simulink library "UXFD_Lib"  (R2016b)
settings: Solver=ode45  StartTime=0.0  StopTime=10.0  RelTol=1e-3  EnableMultiTasking=on
undefined symbols (not defined in the file): BreakpointData, BreakpointData1, BreakpointData2, BreakpointData_One_A, BreakpointData_Two_A, E2E_P01DataIDMode, E2E_P01ReceiverStatusType, EnumClass, iBit, initalValue, No_Runnable_Period, ObB_EidBsgStDerat_C, p_OVERRIDE_MASTER_SWITCH, SlDemoSign, SwitchOff_P, SwitchOn_P, Table, TableData_M, VCCTi33, VSysD_FidVehDerat1_C
libraries: simulink x28, CCMLib x11, UXFD_Lib x8, canmsglib x2, PTCC_Lib x1, hdlsllib x1
(part 7 of 7)

== system UXFD_Lib/Custom/CAN/CanHex2Signed/signal_conditioning ==
  note: 判断输入的BitLength是否（0<u1<=32bit）;
      | 并向下取整。
  In1 : Inport
  Constant1 : Constant  Value=0  OutDataTypeStr=single
      settings: CopyFcn=set_param(gcbh,'ShowName','off');
  Constant2 : Constant  Value=32  OutDataTypeStr=single
      settings: CopyFcn=set_param(gcbh,'ShowName','off');
  Constant4 : Constant  Value=32  OutDataTypeStr=single
      settings: CopyFcn=set_param(gcbh,'ShowName','off');
  Constant7 : Constant  Value=0  OutDataTypeStr=single
      settings: CopyFcn=set_param(gcbh,'ShowName','off');
  Floor : Subsystem  mask(GL_Floor){}
      mask help: Floor block rounds the input variable to the nearest integer towards minus infinity.
      mask init:
      | set_param(gcb,'LinkStatus','none');
      settings: CopyFcn=set_param(gcbh,'ShowName','off');
      mask Display: text(0.1,0.5, 'Floor')
  Relational Operator1 : RelationalOperator  Operator=<  OutDataTypeStr=boolean  RndMeth=Nearest
  Relational Operator2 : RelationalOperator  Operator=>  OutDataTypeStr=boolean  RndMeth=Nearest
  Switch : Switch  Criteria=u2 > Threshold
  Switch1 : Switch  Criteria=u2 > Threshold
  BitLength_BeUsed : Outport
  wires:
  Floor/1(Out1) -> Switch1/1
  Relational Operator2/1 -> Switch/2
  Constant1/1 -> Relational Operator2/2
  Relational Operator1/1 -> Switch1/2
  Switch/1 -> Floor/1(In1), Relational Operator1/1
  Constant4/1 -> Relational Operator1/2
  Constant2/1 -> Switch1/3
  Switch1/1 -> BitLength_BeUsed/1
  Constant7/1 -> Switch/3
  In1/1 -> Relational Operator2/1, Switch/1

== system UXFD_Lib/Custom/CAN/CanHex2Signed/value<0 ==
  hex : Inport
  2^n : Inport  Port=2  OutDataTypeStr=single
  Action Port : ActionPort
  Add : Sum  Inputs=+-
      settings: CopyFcn=set_param(gcbh,'ShowName','off');
  Gain1 : Gain  OutDataTypeStr=single
      settings: CopyFcn=set_param(gcbh,'ShowName','off');
  Gain8 : Gain  OutDataTypeStr=single
      settings: CopyFcn=set_param(gcbh,'ShowName','off');
  Out1 : Outport
  wires:
  Gain1/1 -> Add/2
  2^n/1 -> Gain1/1
  Gain8/1 -> Out1/1
  Add/1 -> Gain8/1
  hex/1 -> Add/1

== system UXFD_Lib/Custom/CAN/CanHex2Signed/value>0 ==
  hex : Inport
  Action Port : ActionPort
  Gain9 : Gain  OutDataTypeStr=single
      settings: CopyFcn=set_param(gcbh,'ShowName','off');
  Out1 : Outport
  wires:
  Gain9/1 -> Out1/1
  hex/1 -> Gain9/1

== system UXFD_Lib/Custom/Diagnose/Dem_SetEventStatus/Dem_SetEventStatus_Enable ==
  EventID : Inport
  EveSt : Inport  Port=2
  Enable : EnablePort
  Dem_SetEventStatus_Asw : S-Function  FunctionName=Dem_SetEventStatus_Asw_SF  SFunctionDeploymentMode=off  EnableBusSupport=off  mask(Legacy Function){SFunctionSpec=void Dem_SetEventStatus_Asw(uint16 u1, uint8 u2), ShowSpec=on}
      mask prompts: ShowSpec "Display function specification"
      mask help:
      | This block allows you to call the legacy functions specified by the following Legacy Code Tool definition:
      | def.SFunctionName = 'Dem_SetEventStatus_Asw_SF';
      | def.OutputFcnSpec = 'void Dem_SetEventStatus_Asw(uint16 u1, uint8 u2)';
      | def.HeaderFiles = {'Dem.h'};
      | def.SourceFiles = {'Dem.c'};
      mask Help: <p>This block was generated automatically by the Legacy Code Tool. For detailed help on this tool, call<a href="matlab:legacy_code('help')"> legacy_code('help')</a>.</p>
      mask Callback ShowSpec:
      | if strcmp(get_param(gcbh, 'ShowSpec'), 'on')
      |   set_param(gcbh, 'MaskDisplay', sprintf('fprintf(''%s'');', get_param(gcbh, 'SFunctionSpec')));
      | else
      |   set_param(gcbh, 'MaskDisplay', sprintf('fprintf(''%s'');', get_param(gcbh, 'FunctionName')));
      | end
      mask Display: fprintf('void Dem_SetEventStatus_Asw(uint16 u1, uint8 u2)');
  wires:
  EveSt/1 -> Dem_SetEventStatus_Asw/2
  EventID/1 -> Dem_SetEventStatus_Asw/1

== system UXFD_Lib/Standard/Discrete dynamics/BumplessRateTransfer/LogicalSwitch1 ==
  In1 : Inport
  In2 : Inport  Port=2
  In3 : Inport  Port=3
  Switch : Switch  Criteria=u2 > Threshold  Threshold=0.5
  Out1 : Outport
  wires:
  In1/1 -> Switch/1
  In3/1 -> Switch/2
  In2/1 -> Switch/3
  Switch/1 -> Out1/1

== system UXFD_Lib/Standard/Discrete dynamics/BumplessRateTransfer/RateLimit ==
  In1 : Inport
  dr : Inport  Port=2
  df : Inport  Port=3
  Abs : Abs
  Add : Sum  Inputs=+-
  Add1 : Sum
  MinMax : MinMax  Function=max  Inputs=2
  MinMax1 : MinMax  Inputs=2
  Product : Product
  Product1 : Product
  Subsystem1 : Subsystem
      mask help:
      | this block use for the situation when the first run use the Initail Value , after the first run , use the CalValue.
      | output is the Initial Value when first run ; otherwise is the calValue.
      mask Display: dpoly([0 0 1], [0 1 0], 'z')
  ts : DataStoreRead  DataStoreName=ts
  y : Outport
  wires:
  In1/1 -> Subsystem1/1(InitialValue), MinMax/1
  Add1/1 -> MinMax1/2
  dr/1 -> Product1/2
  MinMax1/1 -> Subsystem1/2(CalValue), y/1
  Product1/1 -> Add1/2
  MinMax/1 -> MinMax1/1
  Add/1 -> MinMax/2
  Product/1 -> Abs/1
  df/1 -> Product/2
  ts/1 -> Product1/1, Product/1
  Abs/1 -> Add/2
  Subsystem1/1(Output) -> Add1/1, Add/1

== system UXFD_Lib/Standard/Discrete dynamics/BumplessTransfer/LPF1_pole1 ==
  u : Inport
  tc : Inport  Port=2
  Add : Sum  Inputs=-+
  Add1 : Sum
  Constant : Constant  Value=1e-6  OutDataTypeStr=single
  Divide : Product  Inputs=*/
  MinMax : MinMax  Function=max  Inputs=3
  Product : Product
  Subsystem1 : Subsystem
      mask help:
      | this block use for the situation when the first run use the Initail Value , after the first run , use the CalValue.
      | output is the Initial Value when first run ; otherwise is the calValue.
      mask Display: dpoly([0 0 1], [0 1 0], 'z')
  ts : DataStoreRead  DataStoreName=ts
  y : Outport
  wires:
  Add1/1 -> Subsystem1/2(CalValue), y/1
  u/1 -> Subsystem1/1(InitialValue), Add/2
  Add/1 -> Product/1
  MinMax/1 -> Divide/2
  tc/1 -> MinMax/2
  ts/1 -> Divide/1, MinMax/1
  Divide/1 -> Product/2
  Subsystem1/1(Output) -> Add/1, Add1/1
  Product/1 -> Add1/2
  Constant/1 -> MinMax/3

== system UXFD_Lib/Standard/Discrete dynamics/BumplessTransfer/LogicalSwitch1 ==
  In1 : Inport
  In2 : Inport  Port=2
  In3 : Inport  Port=3
  Switch : Switch  Criteria=u2 > Threshold  Threshold=0.5
  Out1 : Outport
  wires:
  In1/1 -> Switch/1
  In3/1 -> Switch/2
  In2/1 -> Switch/3
  Switch/1 -> Out1/1

== system UXFD_Lib/Standard/Discrete dynamics/DLPF1_pole_v2/LogicalSwitch1 ==
  In1 : Inport
  In2 : Inport  Port=2
  In3 : Inport  Port=3
  Switch : Switch  Criteria=u2 > Threshold  Threshold=0.5
  Out1 : Outport
  wires:
  In1/1 -> Switch/1
  In3/1 -> Switch/2
  In2/1 -> Switch/3
  Switch/1 -> Out1/1

== system UXFD_Lib/Standard/Discrete dynamics/HysteresisFilter/Saturation1 ==
  u : Inport
  U : Inport  Port=2
  L : Inport  Port=3
  MinMax : MinMax  Inputs=2
  MinMax1 : MinMax  Function=max  Inputs=2
  y : Outport
  wires:
  L/1 -> MinMax1/2
  MinMax1/1 -> y/1
  u/1 -> MinMax/2
  U/1 -> MinMax/1
  MinMax/1 -> MinMax1/1

== system UXFD_Lib/Standard/Discrete dynamics/LPF1_discreteReset/LogicalSwitch1 ==
  In1 : Inport
  In3 : Inport  Port=2
  In2 : Inport  Port=3
  Switch : Switch  Criteria=u2 ~= 0  Threshold=0.5  SaturateOnIntegerOverflow=on  InputSameDT=on  mask(TL_Switch){data={'logdata',{'maxnumvals',4096,'plotchannels',[]},'output',{'type','Float32'},'date',735300.29228125}}
      settings: CopyFcn=if exist('tl_reset_reviewflag','file')==2,tl_reset_reviewflag(gcbh);end  DeleteFcn=if exist('delete_tlblock','file')==2,delete_tlblock(gcbh);end  NameChangeFcn=if exist('rename_tlblock','file')==2,rename_tlblock(gcbh);end  OpenFcn=if exist('tl_open_blockdlg','file')==2,tl_open_blockdlg(gcbh);else,open_system(gcbh,'parameter');end
      mask Help: eval(['if exist(''tl_online_help'',''file'') == 2, tl_online_help(''Topic'',''TL_Switch''),else, web([''jar:file:///'',matlabroot,''/help/toolbox/simulink/help.jar!/slref/' lower(get_param(gcbh,'Blocktype')) '.html''], ''-helpbrowser''),end'])
      mask Display: plot([-0.05, 1.05, NaN, -0.05, 1.05],[.01, .01, NaN, .99, .99])
  Out1 : Outport
  wires:
  In1/1 -> Switch/1
  In2/1 -> Switch/2
  In3/1 -> Switch/3
  Switch/1 -> Out1/1

== system UXFD_Lib/Standard/Math/Floor/mod1 ==
  In1 : Inport
  In2 : Inport  Port=2
  Mod : Math  Operator=mod  SaturateOnIntegerOverflow=on
  Out1 : Outport
  wires:
  In1/1 -> Mod/1
  Mod/1 -> Out1/1
  In2/1 -> Mod/2

== system UXFD_Lib/Standard/Math/Interpolation/Safe_Divide ==
  In3 : Inport
  In2 : Inport  Port=2
  In1 : Inport  Port=3
  Constant : Constant  Value=0  OutDataTypeStr=Inherit: Inherit via back propagation
  Gain : Gain  Gain=-1
  LogicalSwitch : Subsystem  mask(PAG_Switch_LV1.6_BV2){}
      mask help:
      | Pass through input 1 when input 3 is true;
      | otherwise, pass through input 2
      mask Display:
      | plot([-0.1 0.2 0.2], [0.85 0.85 0.75])
      | plot([-0.1 0.2 0.2], [0.5 0.5 0.6])
      | plot([0.8 1.1], [0.5 0.5])
      | plot([0.15 0.8], [0.6 0.5])
      | plot([-0.1 0.5 0.5], [0.15 0.15 0.6])
  Max : MinMax  Function=max  Inputs=2
  MinMax : MinMax  Inputs=2
  Product1 : Product  Inputs=*/
  Relational Operator : RelationalOperator  Operator=<  OutDataTypeStr=boolean  RndMeth=Nearest
  Out1 : Outport
  wires:
  Constant/1 -> Relational Operator/2
  Relational Operator/1 -> LogicalSwitch/3(In3)
  MinMax/1 -> LogicalSwitch/1(In1)
  In1/1 -> Gain/1, Max/1
  In2/1 -> Relational Operator/1, Max/2, MinMax/1
  Max/1 -> LogicalSwitch/2(In2)
  In3/1 -> Product1/1
  Product1/1 -> Out1/1
  Gain/1 -> MinMax/2
  LogicalSwitch/1(Out1) -> Product1/2

== system UXFD_Lib/Standard/Math/LimitInterpolation/Safe_Divide ==
  In3 : Inport
  In2 : Inport  Port=2
  In1 : Inport  Port=3
  Constant : Constant  Value=0  OutDataTypeStr=Inherit: Inherit via back propagation
  Gain : Gain  Gain=-1
  LogicalSwitch : Subsystem  mask(PAG_Switch_LV1.6_BV2){}
      mask help:
      | Pass through input 1 when input 3 is true;
      | otherwise, pass through input 2
      mask Display:
      | plot([-0.1 0.2 0.2], [0.85 0.85 0.75])
      | plot([-0.1 0.2 0.2], [0.5 0.5 0.6])
      | plot([0.8 1.1], [0.5 0.5])
      | plot([0.15 0.8], [0.6 0.5])
      | plot([-0.1 0.5 0.5], [0.15 0.15 0.6])
  Max : MinMax  Function=max  Inputs=2
  MinMax : MinMax  Inputs=2
  Product1 : Product  Inputs=*/
  Relational Operator : RelationalOperator  Operator=<  OutDataTypeStr=boolean  RndMeth=Nearest
  Out1 : Outport
  wires:
  Constant/1 -> Relational Operator/2
  Relational Operator/1 -> LogicalSwitch/3(In3)
  MinMax/1 -> LogicalSwitch/1(In1)
  In1/1 -> Gain/1, Max/1
  In2/1 -> Relational Operator/1, Max/2, MinMax/1
  Max/1 -> LogicalSwitch/2(In2)
  In3/1 -> Product1/1
  Product1/1 -> Out1/1
  Gain/1 -> MinMax/2
  LogicalSwitch/1(Out1) -> Product1/2

== system UXFD_Lib/Standard/Math/LimitInterpolation/Saturation ==
  u : Inport
  U : Inport  Port=2
  L : Inport  Port=3
  MinMax : MinMax  Inputs=2
  MinMax1 : MinMax  Function=max  Inputs=2
  y : Outport
  wires:
  MinMax/1 -> MinMax1/1
  U/1 -> MinMax/1
  u/1 -> MinMax/2
  MinMax1/1 -> y/1
  L/1 -> MinMax1/2

== system UXFD_Lib/Standard/Math/Round/mod ==
  In1 : Inport
  In2 : Inport  Port=2
  mod : Subsystem  mask(GL_Mod_1.0){}
      mask help: Signed remainder after division.
      mask Display: disp('mod')
  Out1 : Outport
  wires:
  In1/1 -> mod/1(In1)
  mod/1(Out1) -> Out1/1
  In2/1 -> mod/2(In2)

== system UXFD_Lib/Standard/Math/Safe_Divide/LogicalSwitch ==
  In1 : Inport
  In2 : Inport  Port=2
  In3 : Inport  Port=3
  Switch : Switch  Criteria=u2 ~= 0  Threshold=1  OutDataTypeStr=Inherit: Inherit via back propagation  RndMeth=Round  SaturateOnIntegerOverflow=on  InputSameDT=on
      settings: AttributesFormatString=%<Criteria>  CopyFcn=set_param(gcbh,'ShowName','off');
  Out1 : Outport
  wires:
  In1/1 -> Switch/1
  In3/1 -> Switch/2
  In2/1 -> Switch/3
  Switch/1 -> Out1/1

== system UXFD_Lib/Autosar/E2E_P01_Check/E2E_Check/E2E_Check/Data_ID_218 ==
  CheckSum : Inport
  RollingCounter : Inport  Port=2
  AccrPedlNotCmpl_Psd : Inport  Port=3
  AccrPedlNotCmpl_PsdSts : Inport  Port=4
  Data Type Conversion{1..2,4..5} (4 alike) : DataTypeConversion  OutDataTypeStr=uint8
  Data Type Conversion6 : DataTypeConversion
  Mux2 : Mux
  Data_pu8 : Outport
  wires:
  Data Type Conversion4/1 -> Mux2/3
  Data Type Conversion5/1 -> Mux2/4
  Mux2/1 -> Data Type Conversion6/1
  Data Type Conversion6/1 -> Data_pu8/1
  RollingCounter/1 -> Data Type Conversion1/1
  CheckSum/1 -> Data Type Conversion2/1
  AccrPedlNotCmpl_PsdSts/1 -> Data Type Conversion5/1
  AccrPedlNotCmpl_Psd/1 -> Data Type Conversion4/1
  Data Type Conversion1/1 -> Mux2/2
  Data Type Conversion2/1 -> Mux2/1

== system UXFD_Lib/Autosar/E2E_P01_Check/E2E_Check/E2E_Check/E2E_Config_ID_218 ==
  DataLength : Inport
  DataID : Inport  Port=2
  BusCreator2 : BusCreator  Inputs=6  OutDataTypeStr=Bus: E2E_P01ConfigType  NonVirtualBus=on
      settings: CopyFcn=set_param(gcbh,'ShowName','off');  InheritFromInputs=off
  CRCOffset : Constant  Value=0  OutDataTypeStr=uint16
  CounterOffset : Constant  Value=8  OutDataTypeStr=uint16
  DataIDMode : simulink/Sources/Enumerated Constant  OutDataTypeStr=Enum: E2E_P01DataIDMode  Value=E2E_P01DataIDMode.E2E_P01_DATAID_BOTH  SampleTime=inf
  MaxDeltaCounterInit : Constant  Value=14  OutDataTypeStr=uint8
  E2E_Config_ID_218 : Outport
  wires:
  CounterOffset/1 -> BusCreator2/6
  DataLength/1 -> BusCreator2/1
  MaxDeltaCounterInit/1 -> BusCreator2/4
  BusCreator2/1 -> E2E_Config_ID_218/1
  CRCOffset/1 -> BusCreator2/5
  DataID/1 -> BusCreator2/2
  DataIDMode/1 -> BusCreator2/3

== system UXFD_Lib/Autosar/E2E_P01_Check/E2E_Check/E2E_Check/E2E_P01Check_S ==
  ConfigType : Inport
  ReceiverStateType : Inport  Port=2
  Data_pu8 : Inport  Port=3
  S-Function : S-Function  FunctionName=E2E_P01Check_S  SFunctionDeploymentMode=off  EnableBusSupport=off
  Std_ReturnType : Outport
  wires:
  S-Function/1 -> Std_ReturnType/1
  Data_pu8/1 -> S-Function/3
  ConfigType/1 -> S-Function/1
  ReceiverStateType/1 -> S-Function/2

== system UXFD_Lib/Autosar/E2E_P01_Check/E2E_Check/E2E_Check/E2E_P01ReceiverID_218 ==
  AccrPedlNotCmpl_IsUpdated : Inport  OutDataTypeStr=boolean
  Status : Inport  Port=2
  BusCreator3 : BusCreator  Inputs=6  OutDataTypeStr=Bus: E2E_P01ReceiverStateType  NonVirtualBus=on
      settings: CopyFcn=set_param(gcbh,'ShowName','off');  InheritFromInputs=off
  LastValidCounter : Constant  Value=0  OutDataTypeStr=uint8
  LostData : Constant  Value=0  OutDataTypeStr=uint8
  MaxDeltaCounter : Constant  Value=0  OutDataTypeStr=uint8
  WaitForFirstData : Constant  OutDataTypeStr=boolean
  E2E_P01ReceiverState : Outport
  wires:
  LastValidCounter/1 -> BusCreator3/1
  WaitForFirstData/1 -> BusCreator3/3
  MaxDeltaCounter/1 -> BusCreator3/2
  LostData/1 -> BusCreator3/5
  BusCreator3/1 -> E2E_P01ReceiverState/1
  AccrPedlNotCmpl_IsUpdated/1 -> BusCreator3/4
  Status/1 -> BusCreator3/6

== system UXFD_Lib/Custom/CAN/CanHex2Signed/signal_conditioning/Floor ==
  In1 : Inport
  Add : Sum  Inputs=+-
  Constant : Constant  OutDataTypeStr=single
  mod1 : Subsystem  mask(GL_Mod_1.0){}
      mask help: Signed remainder after division.
      mask Display: disp('mod')
  Out1 : Outport
  wires:
  Constant/1 -> mod1/2(In2)
  Add/1 -> Out1/1
  In1/1 -> mod1/1(In1), Add/1
  mod1/1(Out1) -> Add/2

== system UXFD_Lib/Standard/Discrete dynamics/BumplessRateTransfer/RateLimit/Subsystem1 ==
  InitialValue : Inport
  CalValue : Inport  Port=2
  Constant12 : Constant  Value=0
      settings: CopyFcn=set_param(gcbh,'ShowName','off');
  ESubsystem : Subsystem  TreatAsAtomicUnit=on
      mask init:
      | set_param(gcb, 'LinkStatus', 'none');
      mask Display: disp(' ');
  Relational Operator10 : RelationalOperator  Operator===  OutDataTypeStr=boolean  RndMeth=Nearest
      settings: CopyFcn=set_param(gcbh,'ShowName','off');
  Switch1 : Switch  Criteria=u2 ~= 0  Threshold=1  OutDataTypeStr=Inherit: Inherit via back propagation  RndMeth=Round  SaturateOnIntegerOverflow=on  InputSameDT=on
      settings: AttributesFormatString=%<Criteria>  CopyFcn=set_param(gcbh,'ShowName','off');
  Unit Delay : UnitDelay  SampleTime=-1
      settings: CopyFcn=set_param(gcbh,'ShowName','off');
  Unit Delay1 : UnitDelay  SampleTime=-1
      settings: CopyFcn=set_param(gcbh,'ShowName','off');
  Output : Outport
  wires:
  Constant12/1 -> Relational Operator10/2
  ESubsystem/1(Out1) -> Unit Delay/1
  Unit Delay/1 -> Relational Operator10/1
  Relational Operator10/1 -> Switch1/2, ESubsystem/Enable
  InitialValue/1 -> Switch1/1
  CalValue/1 -> Unit Delay1/1
  Switch1/1 -> Output/1
  Unit Delay1/1 -> Switch1/3

== system UXFD_Lib/Standard/Discrete dynamics/BumplessTransfer/LPF1_pole1/Subsystem1 ==
  InitialValue : Inport
  CalValue : Inport  Port=2
  Constant12 : Constant  Value=0
      settings: CopyFcn=set_param(gcbh,'ShowName','off');
  ESubsystem : Subsystem  TreatAsAtomicUnit=on
      mask init:
      | set_param(gcb, 'LinkStatus', 'none');
      mask Display: disp(' ');
  Relational Operator10 : RelationalOperator  Operator===  OutDataTypeStr=boolean  RndMeth=Nearest
      settings: CopyFcn=set_param(gcbh,'ShowName','off');
  Switch1 : Switch  Criteria=u2 ~= 0  Threshold=1  OutDataTypeStr=Inherit: Inherit via back propagation  RndMeth=Round  SaturateOnIntegerOverflow=on  InputSameDT=on
      settings: AttributesFormatString=%<Criteria>  CopyFcn=set_param(gcbh,'ShowName','off');
  Unit Delay : UnitDelay  SampleTime=-1
      settings: CopyFcn=set_param(gcbh,'ShowName','off');
  Unit Delay1 : UnitDelay  SampleTime=-1
      settings: CopyFcn=set_param(gcbh,'ShowName','off');
  Output : Outport
  wires:
  Constant12/1 -> Relational Operator10/2
  ESubsystem/1(Out1) -> Unit Delay/1
  Unit Delay/1 -> Relational Operator10/1
  Relational Operator10/1 -> Switch1/2, ESubsystem/Enable
  InitialValue/1 -> Switch1/1
  CalValue/1 -> Unit Delay1/1
  Switch1/1 -> Output/1
  Unit Delay1/1 -> Switch1/3

== system UXFD_Lib/Standard/Math/Interpolation/Safe_Divide/LogicalSwitch ==
  In1 : Inport
  In2 : Inport  Port=2
  In3 : Inport  Port=3
  Switch : Switch  Threshold=0.5  SaturateOnIntegerOverflow=on  InputSameDT=on  mask(TL_Switch){data={'logdata',{'maxnumvals',4096,'plotchannels',[]},'output',{'type','Float32'},'date',735300.29223627318}}
      settings: CopyFcn=if exist('tl_reset_reviewflag','file')==2,tl_reset_reviewflag(gcbh);end  DeleteFcn=if exist('delete_tlblock','file')==2,delete_tlblock(gcbh);end  NameChangeFcn=if exist('rename_tlblock','file')==2,rename_tlblock(gcbh);end  OpenFcn=if exist('tl_open_blockdlg','file')==2,tl_open_blockdlg(gcbh);else,open_system(gcbh,'parameter');end
      mask Help: eval(['if exist(''tl_online_help'',''file'') == 2, tl_online_help(''Topic'',''TL_Switch''),else, web([''jar:file:///'',matlabroot,''/help/toolbox/simulink/help.jar!/slref/' lower(get_param(gcbh,'Blocktype')) '.html''], ''-helpbrowser''),end'])
      mask Display: plot([-0.05, 1.05, NaN, -0.05, 1.05],[.01, .01, NaN, .99, .99])
  Out1 : Outport
  wires:
  Switch/1 -> Out1/1
  In2/1 -> Switch/3
  In3/1 -> Switch/2
  In1/1 -> Switch/1

== system UXFD_Lib/Standard/Math/LimitInterpolation/Safe_Divide/LogicalSwitch ==
  In1 : Inport
  In2 : Inport  Port=2
  In3 : Inport  Port=3
  Switch : Switch  Threshold=0.5  SaturateOnIntegerOverflow=on  InputSameDT=on  mask(TL_Switch){data={'logdata',{'maxnumvals',4096,'plotchannels',[]},'output',{'type','Float32'},'date',735300.29223627318}}
      settings: CopyFcn=if exist('tl_reset_reviewflag','file')==2,tl_reset_reviewflag(gcbh);end  DeleteFcn=if exist('delete_tlblock','file')==2,delete_tlblock(gcbh);end  NameChangeFcn=if exist('rename_tlblock','file')==2,rename_tlblock(gcbh);end  OpenFcn=if exist('tl_open_blockdlg','file')==2,tl_open_blockdlg(gcbh);else,open_system(gcbh,'parameter');end
      mask Help: eval(['if exist(''tl_online_help'',''file'') == 2, tl_online_help(''Topic'',''TL_Switch''),else, web([''jar:file:///'',matlabroot,''/help/toolbox/simulink/help.jar!/slref/' lower(get_param(gcbh,'Blocktype')) '.html''], ''-helpbrowser''),end'])
      mask Display: plot([-0.05, 1.05, NaN, -0.05, 1.05],[.01, .01, NaN, .99, .99])
  Out1 : Outport
  wires:
  Switch/1 -> Out1/1
  In2/1 -> Switch/3
  In3/1 -> Switch/2
  In1/1 -> Switch/1

== system UXFD_Lib/Standard/Math/Round/mod/mod ==
  In1 : Inport
  In2 : Inport  Port=2
  Mod : Math  Operator=mod  SaturateOnIntegerOverflow=on
  Out1 : Outport
  wires:
  In1/1 -> Mod/1
  Mod/1 -> Out1/1
  In2/1 -> Mod/2

== system UXFD_Lib/Custom/CAN/CanHex2Signed/signal_conditioning/Floor/mod1 ==
  In1 : Inport
  In2 : Inport  Port=2
  Mod : Math  Operator=mod  SaturateOnIntegerOverflow=on
  Out1 : Outport
  wires:
  In1/1 -> Mod/1
  Mod/1 -> Out1/1
  In2/1 -> Mod/2

== system UXFD_Lib/Standard/Discrete dynamics/BumplessRateTransfer/RateLimit/Subsystem1/ESubsystem ==
  Enable_Name : EnablePort
  Constant10 : Constant
      settings: CopyFcn=set_param(gcbh,'ShowName','off');
  Out1 : Outport
  wires:
  Constant10/1 -> Out1/1

== system UXFD_Lib/Standard/Discrete dynamics/BumplessTransfer/LPF1_pole1/Subsystem1/ESubsystem ==
  Enable_Name : EnablePort
  Constant10 : Constant
      settings: CopyFcn=set_param(gcbh,'ShowName','off');
  Out1 : Outport
  wires:
  Constant10/1 -> Out1/1

== stateflow chart UXFD_Lib/Standard/Relation&Logic/Chart ==
